simulink library "ERG_lib"  (R2017a)
settings: Solver=VariableStepAuto  StartTime=0.0  StopTime=10.0  RelTol=1e-3
settings Model: Creator=Admin  LastModifiedBy=Admin

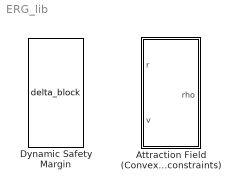
== system ERG_lib ==
  Attraction Field (Convex constraints) : Subsystem  mask{eta=0.0001}
      mask TypeOptions eta: Constant/Value
  Dynamic Safety Margin : M-S-Function  FunctionName=delta_block  Parameters=system_param  mask(Dynamic Safety Margin){system_param=[]}
      mask prompts: system_param "ERGsys object"
      mask help:
      | This block calculates the Dynamic Safety Margin for the system provided in the parameters of the block.
      | NOTE: it is required to compute the Lyapunov functions of the system with the command system_name=system_name.computeQuadraticLyapunov().
      mask Display:
      | port_label('input',1,'x')
      | port_label('input',2,'v')
      | port_label('output',1,'delta')

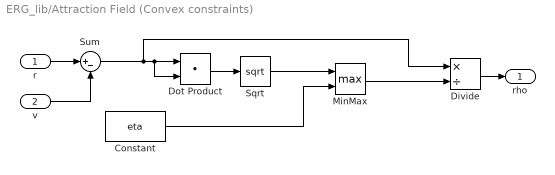
== system ERG_lib/Attraction Field (Convex constraints) ==
  r : Inport
  v : Inport  Port=2
  Constant : Constant  Value=eta
  Divide : Product  Inputs=*/
  Dot Product : DotProduct  InputSameDT=on  OutDataTypeStr=Inherit: Inherit via internal rule
  MinMax : MinMax  Function=max  Inputs=2
  Sqrt : Sqrt  SaturateOnIntegerOverflow=on
  Sum : Sum  Inputs=|+-
  rho : Outport
  wires:
  MinMax/1 -> Divide/2
  Dot Product/1 -> Sqrt/1
  r/1 -> Sum/1
  Sum/1 -> Dot Product/2, Dot Product/1, Divide/1
  v/1 -> Sum/2
  Sqrt/1 -> MinMax/1
  Constant/1 -> MinMax/2
  Divide/1 -> rho/1
